simulink model "model_3"  (R2022a)
settings: Solver=VariableStepAuto  StartTime=0.0  StopTime=3  RelTol=1e-3
values from neighbouring files (symbols this model uses):
  A = [1, -2, 3; 2, -3, 2; -2, 1, -4]    [task_1.m]    (also in task_2.m; task_3.m = [-9, 0, -10; -4, -1, -6; 6, -2, 5]; task_4.m = [-9, 0, -10; -4, -1, -6; 6, -2, 5])
  B = [-3; -1; 3]    [task_1.m]    (also in task_2.m = [3; 1; -1]; task_3.m = [0; 0; 0]; task_4.m = [0; 0; 0])
  C = [0, 0, 0]    [task_1.m]    (also in task_2.m; task_3.m = [2, -1, 2]; task_4.m = [1, 0, 1])
  D = 0    [task_1.m]    (also in task_2.m; task_3.m; task_4.m)
  x_0 = double(inv(Gr_t_1) * integral_f)    [task_3.m]    (also in task_4.m = double(pinv(Gr_t_1) * integral_f))
settings Model: Creator=vital  LastModifiedBy=Family
settings DebuggingCC: UnconnectedInputMsg=warning  UnconnectedOutputMsg=warning  UnconnectedLineMsg=warning
settings RTWCC: DLArmComputeVersion=19.05

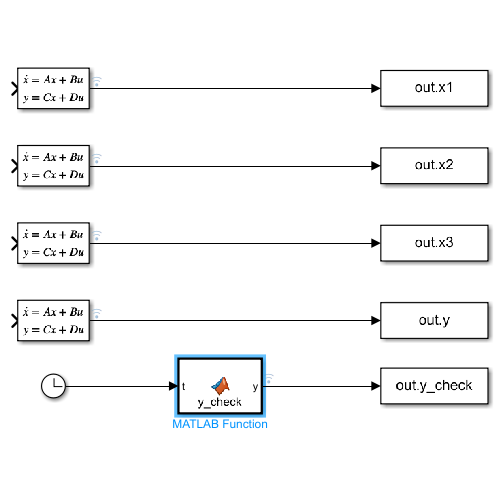
[thumbnail: Simulink's stored preview of the top-level diagram]
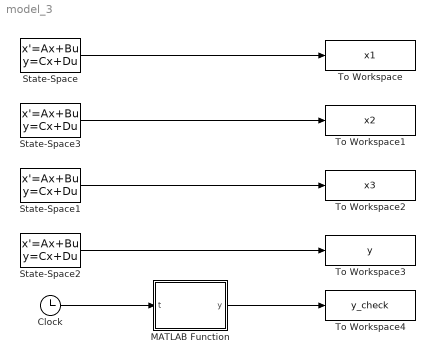
== system model_3 ==
  Clock : Clock
  MATLAB Function : MATLAB Function  TreatAsAtomicUnit=on
  State-Space : StateSpace  A=A  B=B  C=[1, 0, 0]  D=D  InitialCondition=x_0  ContinuousStateAttributes="\"x1\""
  State-Space1 : StateSpace  A=A  B=B  C=[0, 0,1]  D=D  InitialCondition=x_0  ContinuousStateAttributes="\"x3\""
  State-Space2 : StateSpace  A=A  B=B  C=C  D=D  InitialCondition=x_0  ParameterTunability=Unconstrained  ContinuousStateAttributes="\"y\""
  State-Space3 : StateSpace  A=A  B=B  C=[0, 1, 0]  D=D  InitialCondition=x_0  ContinuousStateAttributes="\"x2\""
  To Workspace : ToWorkspace  VariableName=x1  SaveFormat=Timeseries  SampleTime=-1
  To Workspace1 : ToWorkspace  VariableName=x2  SaveFormat=Timeseries  SampleTime=-1
  To Workspace2 : ToWorkspace  VariableName=x3  SaveFormat=Timeseries  SampleTime=-1
  To Workspace3 : ToWorkspace  VariableName=y  SaveFormat=Timeseries  SampleTime=-1
  To Workspace4 : ToWorkspace  VariableName=y_check  SaveFormat=Timeseries  SampleTime=-1
  wires:
  State-Space/1 -> To Workspace/1
  State-Space3/1 -> To Workspace1/1
  State-Space1/1 -> To Workspace2/1
  State-Space2/1 -> To Workspace3/1
  MATLAB Function/1(y) -> To Workspace4/1
  Clock/1 -> MATLAB Function/1(t)

== matlab function model_3/MATLAB Function ==
  data: t input; y output
function y = y_check(t)

y = exp(-3*t)*(-3*cos(2*t) - 2*sin(2*t));
